simulink model "SupervisorFSM_TX"  (R2025b)
settings: configuration reference "MCConfiguration" (kept outside this file)
settings Model: DataDictionary=embeddedBoard_common.sldd  Creator=vvasco  LastModifiedBy=rpumpo
settings ConfigSetRef: SourceName=MCConfiguration

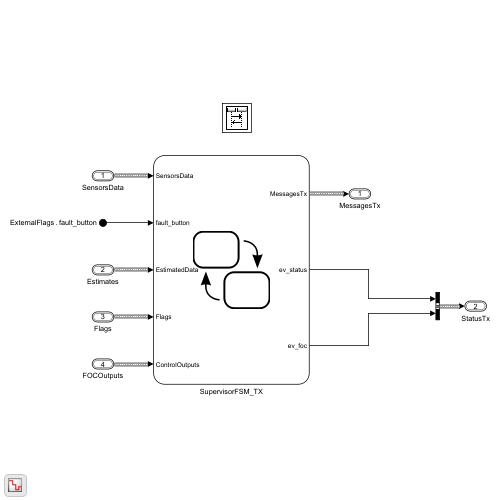
[thumbnail: Simulink's stored preview of the top-level diagram]
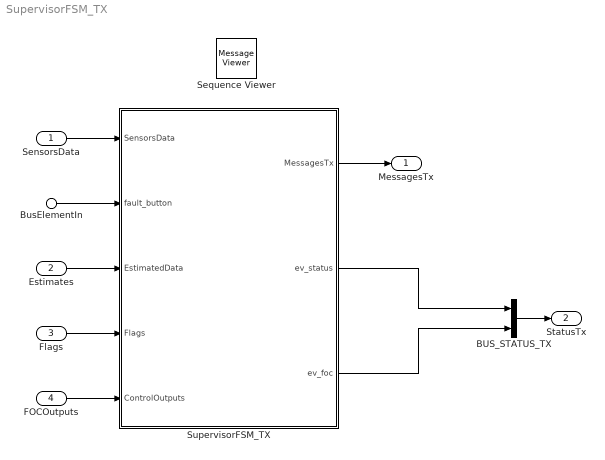
== system SupervisorFSM_TX ==
  SensorsData : Inport  OutDataTypeStr=Bus: SensorsData  BusOutputAsStruct=on
  Estimates : Inport  Port=2  OutDataTypeStr=Bus: EstimatedData  BusOutputAsStruct=on
  Flags : Inport  Port=3  OutDataTypeStr=Bus: Flags  BusOutputAsStruct=on
  FOCOutputs : Inport  Port=4  OutDataTypeStr=Bus: FOCOutputs  BusOutputAsStruct=on
  BusElementIn : Inport  Description=External Fault Button (1 == pressed)  Port=5  PortName=ExternalFlags  Element=fault_button
  BUS_STATUS_TX : BusCreator  Inputs=2  OutDataTypeStr=Bus: BUS_STATUS_TX  NonVirtualBus=on
      settings: InheritFromInputs=off
  Sequence Viewer : MessageViewer  History=1000  SavedRootId=#
  SupervisorFSM_TX : Stateflow chart  TreatAsAtomicUnit=on
  MessagesTx : Outport  OutDataTypeStr=Bus: BUS_MESSAGES_TX  BusOutputAsStruct=on
  StatusTx : Outport  Port=2  OutDataTypeStr=Bus: BUS_STATUS_TX  BusOutputAsStruct=on
  wires:
  SupervisorFSM_TX/1(MessagesTx) -> MessagesTx/1
  SensorsData/1 -> SupervisorFSM_TX/1(SensorsData)
  Flags/1 -> SupervisorFSM_TX/4(Flags)
  BUS_STATUS_TX/1 -> StatusTx/1
  Estimates/1 -> SupervisorFSM_TX/3(EstimatedData)
  FOCOutputs/1 -> SupervisorFSM_TX/5(ControlOutputs)
  BusElementIn/1 -> SupervisorFSM_TX/2(fault_button)
  SupervisorFSM_TX/2(ev_status) -> BUS_STATUS_TX/1
  SupervisorFSM_TX/3(ev_foc) -> BUS_STATUS_TX/2

== stateflow chart SupervisorFSM_TX/SupervisorFSM_TX ==
  settings: updateMethod=DISCRETE  sampleTime=Ts_Supervision  initializeOutput=1
  state MSG_FOC_HANDLER [parallel]
    settings: executionOrder=1
    state Home
    (default) -> MSG_FOC_HANDLER.Home
    MSG_FOC_HANDLER.Home -> MSG_FOC_HANDLER.Home : [Flags.enable_sending_msg_status]
        | {MessagesTx.foc.current = EstimatedData.Iq_filtered;
        | MessagesTx.foc.velocity = EstimatedData.rotor_velocity;
        | MessagesTx.foc.position = SensorsData.motorsensors.qencoder.rotor_angle;
        | ev_foc = true;}
  state MSG_STATUS_HANDLER [parallel]
    settings: executionOrder=2
    state Home
    (default) -> MSG_STATUS_HANDLER.Home
    MSG_STATUS_HANDLER.Home -> MSG_STATUS_HANDLER.Home : [Flags.enable_sending_msg_status]
        | {MessagesTx.status.control_mode = convert(Flags.control_mode);
        | MessagesTx.status.pwm_fbk = ControlOutputs.Vq;
        | MessagesTx.status.flags.ExternalFaultAsserted = fault_button;
        | MessagesTx.status.flags.OverCurrentFailure = Flags.hw_faults.overcurrent;
        | ev_status = true;}
  data: mccontrolmode function_output Enum: MCControlModes size=1; controlmode function_input Enum: ControlModes size=1; MessagesTx output Bus: BUS_MESSAGES_TX; SensorsData input Bus: SensorsData; fault_button input; EstimatedData input Bus: EstimatedData; Flags input Bus: Flags; ControlOutputs input Bus: FOCOutputs; ev_status output boolean; ev_foc output boolean
  function mccontrolmode = convert(controlmode):
    | function mccontrolmode = convert(controlmode)
    | 
    | if controlmode == ControlModes.Idle
    |     mccontrolmode = MCControlModes.Idle;
    | elseif controlmode == ControlModes.Current
    |     mccontrolmode = MCControlModes.Current;
    | elseif controlmode == ControlModes.Velocity
    |     mccontrolmode = MCControlModes.SpeedVoltage;
    | elseif controlmode == ControlModes.Voltage
    |     mccontrolmode = MCControlModes.OpenLoop;
    | elseif controlmode == ControlModes.HwFaultCM
    |     mccontrolmode = MCControlModes.HWFault;
    | elseif controlmode == ControlModes.Position
    |     mccontrolmode = MCControlModes.Position;
    | else
    |     mccontrolmode = MCControlModes.Idle;
    | end
    | 
    | end
